simulink model "practica6"  (R2019b)
settings: Solver=FixedStepAuto  StartTime=0.0  StopTime=10.0  RelTol=1e-3  EnableMultiTasking=on
undefined symbols (not defined in the file): boton, sensor, sonar
libraries: legoev3lib x9
settings Model: ExtModeTrigDuration=2  Creator=alumnopr09  LastModifiedBy=alumnopr09
settings SolverCC: PositivePriorityOrder=on
settings OptimizationCC: EnhancedBackFolding=on  PassReuseOutputArgsAs=Individual arguments  ZeroExternalMemoryAtStartup=off  ZeroInternalMemoryAtStartup=off  MaxStackSize=64  OptimizeBlockOrder=speed  DifferentSizesBufferReuse=on  OptimizationCustomize=off  EfficientTunableParamExpr=on
settings DebuggingCC: ParameterTunabilityLossMsg=error
settings HardwareCC: ProdBitPerPointer=32  ProdBitPerSizeT=32  ProdBitPerPtrDiffT=32  ProdLargestAtomicInteger=Long  ProdWordSize=32  ProdHWDeviceType=ARM Compatible->ARM 9
settings SFSimCC: MATLABDynamicMemAlloc=off
settings RTWCC: SystemTargetFile=ert.tlc  HardwareBoard=LEGO MINDSTORMS EV3  TLCOptions="-aInlineSetEventsForThisBaseRateFcn=TLC_FALSE -aSuppressMultiTaskScheduler=TLC_FALSE  -aRateBasedStepFcn=0"  TemplateMakefile=ert_default_tmf  GenerateReport=on  Toolchain=Sourcery G++ Lite v2009q3  IncludeHyperlinkInReport=on  LaunchReport=on  GenerateTraceInfo=on  GenerateTraceReport=on  GenerateTraceReportSl=on  GenerateTraceReportSf=on  GenerateTraceReportEml=on
settings CodeAppCC: ForceParamTrailComments=on  IgnoreCustomStorageClasses=off  OperatorAnnotations=on  SimulinkDataObjDesc=on  SFDataObjDesc=on  InsertBlockDesc=on
settings ERTTargetCC: SupportContinuousTime=on  SupportVariableSizeSignals=on

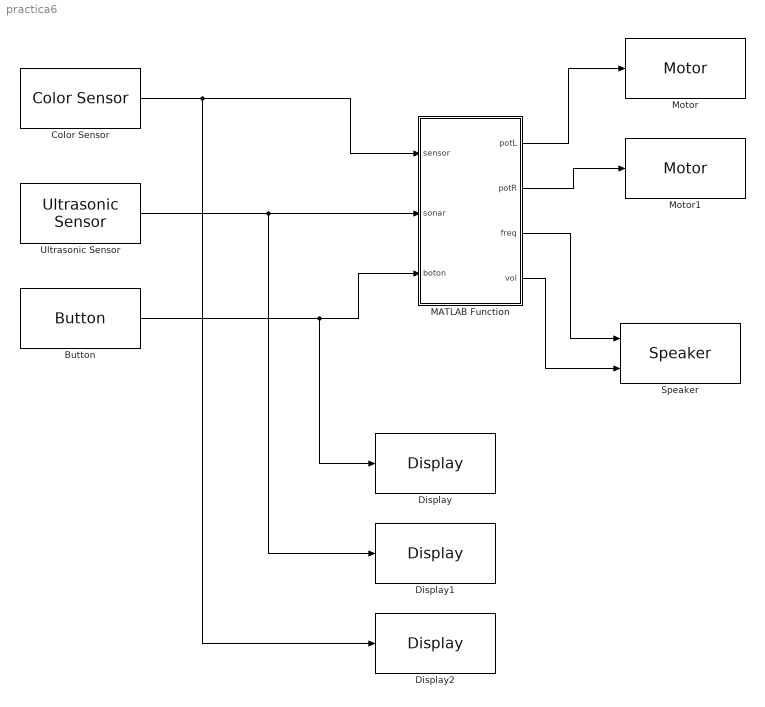
== system practica6 ==
  Button : legoev3lib/Button  buttonType=Up  sampleTime=0.1
      settings: SourceProductName=Simulink Support Package for LEGO MINDSTORMS EV3 Hardware  SourceProductBaseCode=LEGOEV3
  Color Sensor : legoev3lib/Color Sensor  portNumber=4  mode=Reflected light intensity  sampleTime=0.1
      settings: SourceProductName=Simulink Support Package for LEGO MINDSTORMS EV3 Hardware  SourceProductBaseCode=LEGOEV3
  Display : legoev3lib/Display  slcdStr=boton:  slcdLine=1  slcdFormat=Decimal
      settings: SourceProductName=Simulink Support Package for LEGO MINDSTORMS EV3 Hardware  SourceProductBaseCode=LEGOEV3
  Display1 : legoev3lib/Display  slcdStr=sonar:  slcdLine=2  slcdFormat=Decimal
      settings: SourceProductName=Simulink Support Package for LEGO MINDSTORMS EV3 Hardware  SourceProductBaseCode=LEGOEV3
  Display2 : legoev3lib/Display  slcdStr=sensor:  slcdLine=3  slcdFormat=Decimal
      settings: SourceProductName=Simulink Support Package for LEGO MINDSTORMS EV3 Hardware  SourceProductBaseCode=LEGOEV3
  MATLAB Function : MATLAB Function  TreatAsAtomicUnit=on
  Motor : legoev3lib/Motor  sportNumber=D  sstopAction=Brake
  Motor1 : legoev3lib/Motor  sportNumber=A  sstopAction=Brake
  Speaker : legoev3lib/Speaker  sinputMode=Frequency and volume  sspeakerFreq=100  sspeakerVolume=50  sspeakerDuration=100
      settings: SourceProductName=Simulink Support Package for LEGO MINDSTORMS EV3 Hardware  SourceProductBaseCode=LEGOEV3
  Ultrasonic Sensor : legoev3lib/Ultrasonic Sensor  PortNumber=1  sampleTime=0.1
      settings: SourceProductName=Simulink Support Package for LEGO MINDSTORMS EV3 Hardware  SourceProductBaseCode=LEGOEV3
  wires:
  Ultrasonic Sensor/1 -> Display1/1, MATLAB Function/2(sonar)
  Color Sensor/1 -> Display2/1, MATLAB Function/1(sensor)
  Button/1 -> Display/1, MATLAB Function/3(boton)
  MATLAB Function/1(potL) -> Motor/1
  MATLAB Function/2(potR) -> Motor1/1
  MATLAB Function/3(freq) -> Speaker/1
  MATLAB Function/4(vol) -> Speaker/2

== matlab function practica6/MATLAB Function ==
  data: sensor input; potL output; sonar input; boton input; potR output; freq output; vol output
function [potL, potR, freq, vol] = main(sensor, sonar, boton)
p = 50; % potencia motores
freq=0; % in Hz
vol=0; % from 0 to 100
potL=0; % pot motor izq
potR=0; % pot motor der

% estado = true --> buscar
% estado = false --> parado
persistent estado 
if (isempty(estado))
    estado = true;
end

if (estado) % Estoy buscando
    % Compruebo si veo un papel
    detected = Foraging(sensor);
    if (detected) % Detecto algo
        estado = false; 
    else % Sigo sin ver nada
        % Compruebo si tengo obstaculo
        [ignore, pl, pr] = ObstacleAvoidance(sonar,p);
        if (ignore) % Deambulamos
            % Movimientos aleatorios
            [pl, pr] = Wandering(p, randi([1,100],[1,1]));      
        end
        potL = pl;
        potR = pr;
        estado = true; % Redundante

    end    
else % he encontrado algo
    freq = 528; % in Hz
    vol=20; % from 0 to 100
    % boton = 0 --> Not pressed
    % boton = 1 --> Pressed
    if (boton)
        estado = true;
    end
end

%-------------------------------
% Estado del robot y del altavoz
%-------------------------------
function detected = Foraging(sensor)
umbral_luz = 50;

if (sensor > umbral_luz) % ha encontrado un objeto
    detected = true;
    
else % no he encontrado nada
    detected = false;
end

%-----------------------------------
% Deteccion obstaculos y pot motores
%-----------------------------------
function [ignore, pl, pr] = ObstacleAvoidance(sonar,p)
umbral_dist = 35; %cm

if (sonar < umbral_dist) 
   pl = -p; 
   pr = -20;
   ignore = false;
else 
   ignore = true;
   pl=0;
   pr=0;
end

%---------------------------------
% Movimientos aleatorios del robot
%---------------------------------
function [pl, pr] = Wandering(p, n_iteraciones)
pl_backup = p;
pr_backup = p;
if (n_iteraciones < 20) %Giro der
   pl_backup = randi([-p,p],[1,1]);
   pr_backup = -pl_backup; 
elseif (n_iteraciones < 40) %Giro izq
   pr_backup = randi([-p,p],[1,1]);
   pl_backup = -pr_backup; 
end 
pl = pl_backup;
pr = pr_backup;
